simulink model "T3_SIM_COPIE_1"  (R2023b)
settings: Solver=VariableStepAuto  StartTime=0.0  StopTime=75  RelTol=1e-3
undefined symbols (not defined in the file): B1, B2, B_p1, B_p2, B_phi, B_psi, C1, C2, C_phi, C_psi, D_p1, D_p2, g, I1, I2, I_phi, I_psi, K1, K2, K_b1, K_b2, K_gyro, K_i1, K_i2, K_omega1, K_omega2, l, m, R1, R2
settings Model: Creator=Mihai Dinu  LastModifiedBy=Mihai Dinu
settings ModelReferenceCC: EnableRefExpFcnMdlSchedulingChecks=on

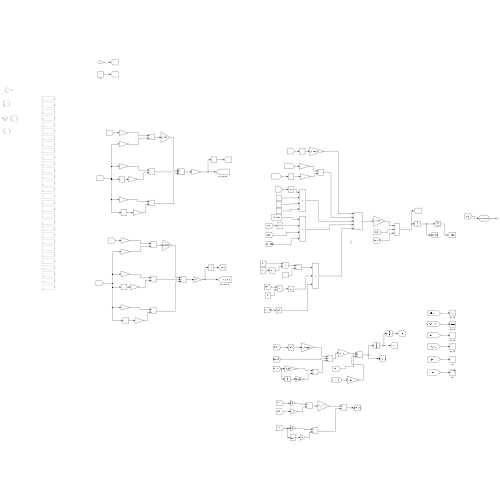
[thumbnail: Simulink's stored preview of the top-level diagram]
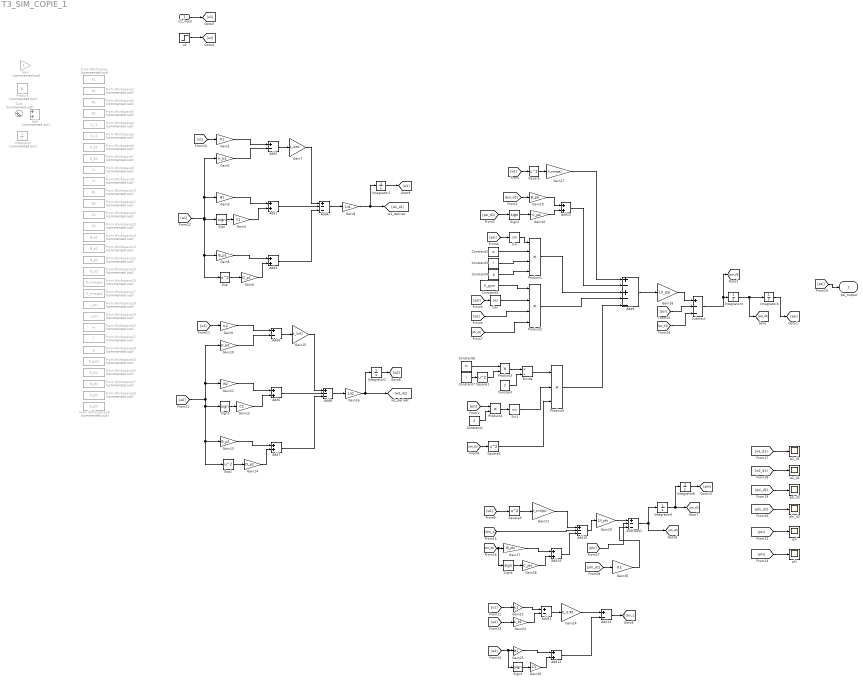
== system T3_SIM_COPIE_1 ==
  u1_input : Inport
  Add : Sum  Commented=on
  Add{1,3,5,7,10,12,14} (7 alike) : Sum
  Add{2,6,11,13} (4 alike) : Sum  Inputs=+-
  Add15 : Sum  Inputs=+--
  Add4 : Sum  Inputs=+--
  Add8 : Sum  Inputs=+--
  Add9 : Sum  Inputs=+-+--
  Constant : Constant  Value=2
  Constant1 : Constant  Value=2
  Constant2 : Constant  Value=m
  Constant3 : Constant  Value=l
  Constant4 : Constant  Value=g
  Constant5 : Constant  Value=K_gyro
  Constant6 : Constant  Value=m
  Constant7 : Constant  Value=l
  Cos : Trigonometry  Operator=cos
  Divide : Product  Inputs=*/
  Exp : Math  Operator=square
  Exp1 : Math  Operator=square
  From Workspace : FromWorkspace  Commented=on  VariableName=K1
  From Workspace1 : FromWorkspace  Commented=on  VariableName=K2
  From Workspace10 : FromWorkspace  Commented=on  VariableName=B1
  From Workspace11 : FromWorkspace  Commented=on  VariableName=B2
  From Workspace12 : FromWorkspace  Commented=on  VariableName=C1
  From Workspace13 : FromWorkspace  Commented=on  VariableName=C2
  From Workspace14 : FromWorkspace  Commented=on  VariableName=B_p1
  From Workspace15 : FromWorkspace  Commented=on  VariableName=B_p2
  From Workspace16 : FromWorkspace  Commented=on  VariableName=K_omega1
  From Workspace17 : FromWorkspace  Commented=on  VariableName=K_omega2
  From Workspace18 : FromWorkspace  Commented=on  VariableName=I_psi
  From Workspace19 : FromWorkspace  Commented=on  VariableName=I_phi
  From Workspace2 : FromWorkspace  Commented=on  VariableName=R1
  From Workspace20 : FromWorkspace  Commented=on  VariableName=m
  From Workspace21 : FromWorkspace  Commented=on  VariableName=l
  From Workspace22 : FromWorkspace  Commented=on  VariableName=D_p1
  From Workspace23 : FromWorkspace  Commented=on  VariableName=D_p2
  From Workspace24 : FromWorkspace  Commented=on  VariableName=g
  From Workspace25 : FromWorkspace  Commented=on  VariableName=K_gyro
  From Workspace26 : FromWorkspace  Commented=on  VariableName=B_psi
  From Workspace27 : FromWorkspace  Commented=on  VariableName=B_phi
  From Workspace28 : FromWorkspace  Commented=on  VariableName=C_psi
  From Workspace29 : FromWorkspace  Commented=on  VariableName=C_phi
  From Workspace3 : FromWorkspace  Commented=on  VariableName=R2
  From Workspace4 : FromWorkspace  Commented=on  VariableName=K_i1
  From Workspace5 : FromWorkspace  Commented=on  VariableName=K_i2
  From Workspace6 : FromWorkspace  Commented=on  VariableName=K_b1
  From Workspace7 : FromWorkspace  Commented=on  VariableName=K_b2
  From Workspace8 : FromWorkspace  Commented=on  VariableName=I1
  From Workspace9 : FromWorkspace  Commented=on  VariableName=I2
  Gain : Gain  Commented=on
  Gain1 : Gain  Gain=K1
  Gain10 : Gain  Gain=K_b2
  Gain11 : Gain  Gain=B2
  Gain12 : Gain  Gain=C2
  Gain13 : Gain  Gain=B_p2
  Gain14 : Gain  Gain=D_p2
  Gain15 : Gain  Gain=K_i2/R2
  Gain16 : Gain  Gain=1/I2
  Gain17 : Gain  Gain=K_omega1
  Gain18 : Gain  Gain=1/I_psi
  Gain19 : Gain  Gain=B_psi
  Gain2 : Gain  Gain=K_b1
  Gain20 : Gain  Gain=C_psi
  Gain21 : Gain  Gain=K_omega2
  Gain22 : Gain  Gain=K1
  Gain23 : Gain  Gain=K_b1
  Gain24 : Gain  Gain=K_i1/R1
  Gain25 : Gain  Gain=B1
  Gain26 : Gain  Gain=C1
  Gain27 : Gain  Gain=B_phi
  Gain28 : Gain  Gain=C_phi
  Gain29 : Gain  Gain=1/I_phi
  Gain3 : Gain  Gain=B1
  Gain30 : Gain  Gain=0.1
  Gain4 : Gain  Gain=C1
  Gain5 : Gain  Gain=B_p1
  Gain6 : Gain  Gain=D_p1
  Gain7 : Gain  Gain=K_i1/R1
  Gain8 : Gain  Gain=1/I1
  Gain9 : Gain  Gain=K2
  Integrator : Integrator  Commented=on
  Integrator{1..6} (6 alike) : Integrator
  Product : Product  Commented=on
  Product1 : Product  Inputs=4
  Product2 : Product  Inputs=4
  Product3 : Product
  Product4 : Product
  Product5 : Product  Inputs=3
  Sign{,1..4} (5 alike) : Signum
  Sin : Trigonometry
  Sin1 : Trigonometry
  Square{,1..3} (4 alike) : Math  Operator=square
  Subtract : Sum  Inputs=+--
  Subtract1 : Sum  Inputs=+--
  Sum : Sum  Commented=on  Inputs=|++
  phi : Scope
  phi_d2 : Scope
  psi : Scope
  psi_d2 : Scope
  u2 : Step  SampleTime=0
  w1_d1 : Scope
  w2_d2 : Scope
  psi_output : Outport  SignalName=psi_output
  wires:
  Sign/1 -> Gain4/1
  Gain3/1 -> Add1/1
  Gain4/1 -> Add1/2
  Gain1/1 -> Add2/1
  Gain2/1 -> Add2/2
  Exp/1 -> Gain6/1
  Gain5/1 -> Add3/1
  Gain6/1 -> Add3/2
  Add2/1 -> Gain7/1
  Gain7/1 -> Add4/1
  Add1/1 -> Add4/2
  Add3/1 -> Add4/3
  Add4/1 -> Gain8/1
  Gain8/1 -> [w1_d1], Integrator1/1
  Sign1/1 -> Gain12/1
  Gain9/1 -> Add6/1
  Gain16/1 -> [w2_d1], Integrator2/1
  Exp1/1 -> Gain14/1
  [u2] -> Gain9/1
  Gain13/1 -> Add7/1
  Gain11/1 -> Add5/1
  Gain15/1 -> Add8/1
  Add8/1 -> Gain16/1
  Add6/1 -> Gain15/1
  Add5/1 -> Add8/2
  Add7/1 -> Add8/3
  Gain10/1 -> Add6/2
  Gain14/1 -> Add7/2
  Gain12/1 -> Add5/2
  [w1] -> Square/1
  Square/1 -> Gain17/1
  Gain17/1 -> Add9/1
  Integrator3/1 -> [psi_d1], Integrator4/1
  Integrator4/1 -> [psi]
  Gain18/1 -> Subtract/1
  [psi_d1] -> Gain19/1
  [psi_d1] -> Sign2/1
  Sign2/1 -> Gain20/1
  Gain19/1 -> Add10/1
  Gain20/1 -> Add10/2
  [psi] -> Sin/1
  Sin/1 -> Product1/1
  Constant2/1 -> Product1/2
  Constant3/1 -> Product1/3
  Constant4/1 -> Product1/4
  [psi] -> Cos/1
  Constant5/1 -> Product2/1
  Cos/1 -> Product2/2
  [w1] -> Product2/3
  [phi_d1] -> Product2/4
  Product3/1 -> Divide/1
  Constant/1 -> Divide/2
  [psi] -> Product4/1
  Constant1/1 -> Product4/2
  Product4/1 -> Sin1/1
  [phi_d1] -> Square2/1
  Divide/1 -> Product5/1
  Sin1/1 -> Product5/2
  Square2/1 -> Product5/3
  Add10/1 -> Add9/2
  Product1/1 -> Add9/3
  Product2/1 -> Add9/4
  Product5/1 -> Add9/5
  Add9/1 -> Gain18/1
  [w2] -> Square3/1
  Square3/1 -> Gain21/1
  u1_input/1 -> [u1]
  [u1] -> Gain1/1
  u2/1 -> [u2]
  [u1] -> Gain22/1
  [w1] -> Gain23/1
  Gain22/1 -> Add11/1
  Gain23/1 -> Add11/2
  Add11/1 -> Gain24/1
  [w1] -> Sign3/1, Gain25/1
  Sign3/1 -> Gain26/1
  Gain25/1 -> Add12/1
  Gain26/1 -> Add12/2
  Add12/1 -> Add13/2
  Gain24/1 -> Add13/1
  Add13/1 -> [tau_c]
  [phi_d1] -> Sign4/1, Gain27/1
  Sign4/1 -> Gain28/1
  Gain28/1 -> Add14/2
  Gain27/1 -> Add14/1
  Gain21/1 -> Add15/1
  [tau_c] -> Add15/2
  Add14/1 -> Add15/3
  Add15/1 -> Gain29/1
  Integrator5/1 -> Integrator6/1, [phi_d1]
  [w1_d1] -> w1_d1/1
  [w2_d1] -> w2_d2/1
  [phi_d2] -> phi_d2/1
  [psi_d2] -> psi_d2/1
  Integrator2/1 -> [w2]
  [w2] -> Exp1/1, Gain13/1, Sign1/1, Gain11/1, Gain10/1
  Integrator1/1 -> [w1]
  [w1] -> Exp/1, Gain5/1, Sign/1, Gain3/1, Gain2/1
  Constant6/1 -> Product3/1
  Constant7/1 -> Square1/1
  [psi] -> psi/1
  [phi] -> phi/1
  Integrator6/1 -> [phi]
  Square1/1 -> Product3/2
  Subtract/1 -> [psi_d2], Integrator3/1
  [psi] -> Subtract/2
  [psi_d1] -> Subtract/3
  [phi_d1] -> Gain30/1
  Gain30/1 -> Subtract1/3
  [phi] -> Subtract1/2
  Gain29/1 -> Subtract1/1
  Subtract1/1 -> [phi_d2], Integrator5/1
  [psi] -> psi_output/1
